simulink model "DvrSimKeybdCircuit_cs"  (R2016a)
settings: Solver=ode5  SolverMode=SingleTasking  StartTime=0.0  StopTime=inf  FixedStep=1/1000  RelTol=1e-3
PreLoadFcn:
  | mbxruntime.callbacks.PreLoadFcn(bdroot);
PostLoadFcn:
  | mbxruntime.callbacks.PostLoadFcn(bdroot);
InitFcn:
  | mbxruntime.callbacks.InitFcn(bdroot);
StartFcn:
  | mbxruntime.callbacks.StartFcn(bdroot);
StopFcn:
  | mbxruntime.callbacks.StopFcn(bdroot);
model workspace (MAT data in the model file):
  mbox_table : struct (value not decoded)
  model_closed = 0
  sim_status = 0
undefined symbols (not defined in the file or in its folder): BMotor1, BMotor2, BrkDelayTime, DControlB, Delay1, Delay2, DiscIntNeverNeededParam, IControlB, JMotor1, JMotor2, PControlB, PreScanCarSimLoadFcn, ratioGearF, ratioGearR, TorqDelayTime, Tstep
undefined symbols (not defined in the file): SteeringColumn, SteeringWheel, WheelL0, WheelL1, WheelR0, WheelR1
libraries: simulink x12, simulink_extras x5, MyLib x3, PreScanSimulinkLibrary x3, Solver_SF x2, pil_lib x1, PreScanUsefulBlocks x1
(part 3 of 9)

== system DvrSimKeybdCircuit_cs/Roewe_550_S_Sedan_1/Subsystem1 ==
  CarSimOut : Inport
  Bus Selector : BusSelector  OutputSignals=SprungMass_Pos_Global_x[m] (signal 1),SprungMass_Pos_Global_y[m] (signal 2),SprungMass_Pos_Global_z[m] (signal 3),VehicleCoG_Vx[km/h] (signal 4),VehicleCoG_Vy[km/h] (signal 5),VehicleCoG_Vz[km/h] (signal 6),SprungMass_Angle_Global_Roll[deg] (signal 7),SprungMass_Angle_Global_Pitch[deg] (signal 8),SprungMass_Angle_Global_Yaw[deg] (signal 9),CarSim_Pos_Wheel_FL_x[m] (signal 10),CarSim_Pos_Wheel_FL_y[m] (signal 11),CarSim_Pos_Wheel_FL_z[m] (signal 12),CarSim_Pos_Wheel_FR_x[m] (signal 13),CarSim_Pos_Wheel_FR_y[m] (signal 14),CarSim_Pos_Wheel_FR_z[m] (signal 15),CarSim_Pos_Wheel_RL_x[m] (signal 16),CarSim_Pos_Wheel_RL_y[m] (signal 17),CarSim_Pos_Wheel_RL_Z[m] (signal 18),CarSim_Pos_Wheel_RR_x[m] (signal 19),CarSim_Pos_Wheel_RR_y[m] (signal 20),CarSim_Pos_Wheel_RR_z[m] (signal 21),CarSim_Angle_Wheel_FL_Roll[deg] (signal 22),CarSim_Angle_Wheel_FL_Rot[rev] (signal 23),CarSim_Angle_Wheel_FL_Steer[deg] (signal 24),CarSim_Angle_Wheel_FR_Roll[deg] (signal 25),CarSim_Angle_Wheel_FR_Rot[rev] (signal 26),CarSim_Angle_Wheel_FR_Steer[deg] (signal 27),CarSim_Angle_Wheel_RL_Roll[deg] (signal 28),CarSim_Angle_Wheel_RL_Rot[rev] (signal 29),CarSim_Angle_Wheel_RL_Steer[deg] (signal 30),CarSim_Angle_Wheel_RR_Roll[deg] (signal 31),CarSim_Angle_Wheel_RR_Rot[rev] (signal 32),CarSim_Angle_Wheel_RR_Steer[deg] (signal 33),SteeringWheelAngle[deg] (signal 34),Axle1ReducedSW (signal 35)
  CarSim2PreScanSTATE : Subsystem  Tag=CarSim2PreScanSTATE  mask(CarSim2PreScan:){z0=0.53}
      mask prompts: z0 "PreScan Actor initial COG z-position wrt GLOBAL axis system [m]"
      mask help: This block converts the outputs coming from the CarSim block into consistent PreScan signals.
  CarSim2PreScan_BUS : Subsystem  Tag=CarSim2PreScan_BUS  mask(PreScan block: CarSim to PreScan BUS){TyreRadius=0.44999998807907104, cogZOffset=0}
      mask prompts: TyreRadius "Tyre Radius [m]"; cogZOffset "cog Z offset [m]"
      mask help: CarSim to PreScan BUS selector
      mask Help: eval('openHelp()')
      mask Display: disp('PreScan BUS\nVehicleDynamics')
  CarSim2PreScan_ContactAdapter : Subsystem  Tag=CarSim2PreScan_ContactAdapter  mask{wheelRadius=0.44999998807907104}
      mask prompts: wheelRadius "Wheel radius:"
  Demux : Demux  Outputs=[18 -1]
  Mux : Mux  Inputs=35
  MuxState1 : Subsystem  Tag=mux/State  mask(Empty Dynamics State Block){positioningmode=on, TimeStep=1/1000}
      mask prompts: positioningmode "Positioning Mode"; TimeStep "Auto Assigned: Time Step [s]"
      mask help:
      | Build the state of an actor based on user input.
      | The user can either use positioning mode or dynamics mode.
      | - When using positioning mode the position and orientation of the actor are set directly based on the input. Expected input is relative to the initial position and orientation of the actor. It's also possible to specify the velocity of the actor, though this input isn't used, only passed on.
      | - When using dynamics mode the position input is ignored. Expected input is velocity and orientation. The velocity is relative the current orientation of the actor, while orientation is relative to its initial orientation. The position of the actor is calculated based on the velocity and orientation given.
      settings: DeleteFcn=PreScanBlockDeleteFcn;
  Scope : Scope
  Terminator_1 : Terminator
  State : Outport
  State_BUS : Outport  Port=2
  ContactParams : Outport  Port=3
  wires:
  CarSimOut/1 -> Bus Selector/1
  Bus Selector/4 -> Mux/4  "<VehicleCoG_Vx[km/h] (signal 4)>"
  Bus Selector/1 -> Mux/1  "<SprungMass_Pos_Global_x[m] (signal 1)>"
  Bus Selector/2 -> Mux/2  "<SprungMass_Pos_Global_y[m] (signal 2)>"
  Bus Selector/3 -> Mux/3  "<SprungMass_Pos_Global_z[m] (signal 3)>"
  Bus Selector/24 -> Mux/24  "<CarSim_Angle_Wheel_FL_Steer[deg] (signal 24)>"
  Bus Selector/28 -> Mux/28  "<CarSim_Angle_Wheel_RL_Roll[deg] (signal 28)>"
  Bus Selector/11 -> Mux/11  "<CarSim_Pos_Wheel_FL_y[m] (signal 11)>"
  Bus Selector/10 -> Mux/10  "<CarSim_Pos_Wheel_FL_x[m] (signal 10)>"
  Bus Selector/7 -> Mux/7  "<SprungMass_Angle_Global_Roll[deg] (signal 7)>"
  Bus Selector/26 -> Mux/26  "<CarSim_Angle_Wheel_FR_Rot[rev] (signal 26)>"
  Bus Selector/30 -> Mux/30  "<CarSim_Angle_Wheel_RL_Steer[deg] (signal 30)>"
  Bus Selector/31 -> Mux/31  "<CarSim_Angle_Wheel_RR_Roll[deg] (signal 31)>"
  Bus Selector/16 -> Mux/16  "<CarSim_Pos_Wheel_RL_x[m] (signal 16)>"
  Bus Selector/6 -> Mux/6  "<VehicleCoG_Vz[km/h] (signal 6)>"
  Bus Selector/12 -> Mux/12  "<CarSim_Pos_Wheel_FL_z[m] (signal 12)>"
  Bus Selector/21 -> Mux/21  "<CarSim_Pos_Wheel_RR_z[m] (signal 21)>"
  Bus Selector/27 -> Mux/27  "<CarSim_Angle_Wheel_FR_Steer[deg] (signal 27)>"
  Bus Selector/5 -> Mux/5  "<VehicleCoG_Vy[km/h] (signal 5)>"
  Bus Selector/19 -> Mux/19  "<CarSim_Pos_Wheel_RR_x[m] (signal 19)>"
  Bus Selector/23 -> Mux/23  "<CarSim_Angle_Wheel_FL_Rot[rev] (signal 23)>"
  Bus Selector/32 -> Mux/32  "<CarSim_Angle_Wheel_RR_Rot[rev] (signal 32)>"
  Bus Selector/29 -> Mux/29  "<CarSim_Angle_Wheel_RL_Rot[rev] (signal 29)>"
  Bus Selector/35 -> Mux/35  "<Axle1ReducedSW (signal 35)>"
  Bus Selector/13 -> Mux/13  "<CarSim_Pos_Wheel_FR_x[m] (signal 13)>"
  Bus Selector/34 -> Mux/34  "<SteeringWheelAngle[deg] (signal 34)>"
  Bus Selector/9 -> Mux/9  "<SprungMass_Angle_Global_Yaw[deg] (signal 9)>"
  Bus Selector/20 -> Mux/20  "<CarSim_Pos_Wheel_RR_y[m] (signal 20)>"
  Bus Selector/25 -> Mux/25  "<CarSim_Angle_Wheel_FR_Roll[deg] (signal 25)>"
  Bus Selector/8 -> Mux/8  "<SprungMass_Angle_Global_Pitch[deg] (signal 8)>"
  Bus Selector/15 -> Mux/15  "<CarSim_Pos_Wheel_FR_z[m] (signal 15)>"
  Bus Selector/17 -> Mux/17  "<CarSim_Pos_Wheel_RL_y[m] (signal 17)>"
  Bus Selector/18 -> Mux/18  "<CarSim_Pos_Wheel_RL_Z[m] (signal 18)>"
  Bus Selector/14 -> Mux/14  "<CarSim_Pos_Wheel_FR_y[m] (signal 14)>"
  Bus Selector/22 -> Mux/22  "<CarSim_Angle_Wheel_FL_Roll[deg] (signal 22)>"
  Bus Selector/33 -> Mux/33  "<CarSim_Angle_Wheel_RR_Steer[deg] (signal 33)>"
  Mux/1 -> CarSim2PreScan_BUS/1(CarSim_In), Demux/1
  MuxState1/1(state) -> CarSim2PreScan_ContactAdapter/1(State), State/1
  CarSim2PreScanSTATE/1(x [m]) -> MuxState1/1(x [m])
  CarSim2PreScanSTATE/2(y [m]) -> MuxState1/2(y [m])
  CarSim2PreScanSTATE/3(z [m]) -> Scope/1, MuxState1/3(z [m])
  CarSim2PreScanSTATE/4(dx [m/s]) -> MuxState1/4(dx [m/s])
  CarSim2PreScanSTATE/5(dy [m/s]) -> MuxState1/5(dy [m/s])
  CarSim2PreScanSTATE/6(dz [m/s]) -> MuxState1/6(dz [m/s])
  CarSim2PreScanSTATE/7(R [rad]) -> MuxState1/7(R [rad])
  CarSim2PreScanSTATE/8(P [rad]) -> MuxState1/8(P [rad])
  CarSim2PreScanSTATE/9(Y [rad]) -> MuxState1/9(Y [rad])
  CarSim2PreScan_BUS/1(PreScanBUS_VehicleDynamics) -> CarSim2PreScan_ContactAdapter/2(State_Bus), State_BUS/1
  CarSim2PreScan_ContactAdapter/1(ContactParams) -> ContactParams/1
  Demux/1 -> CarSim2PreScanSTATE/1(CarSim_In)
  Demux/2 -> Terminator_1/1

== system DvrSimKeybdCircuit_cs/Roewe_550_S_Sedan_1/TIS_1_StandardCoh_Demux ==
  TIS : Inport
  Bus Creator : BusCreator  Inputs=16
  Bus Selector : BusSelector  OutputSignals=ActiveBeamID[-],Range[m],DopplerVelocity[ms-1],DopplerVelocityX[ms-1],DopplerVelocityY[ms-1],DopplerVelocityZ[ms-1],Theta[deg],Phi[deg],TargetID[-],TargetTypeID[-],DopplerVelocityTranslationX[ms-1],DopplerVelocityTranslationY[ms-1],DopplerVelocityTranslationZ[ms-1],DopplerVelocityRotationX[ms-1],DopplerVelocityRotationY[ms-1],DopplerVelocityRotationZ[ms-1]
  ScannerSensorLegacyBusConversion : PreScanUsefulBlocks/ScannerSensorLegacyBusConversion  MAXMESSAGES=MAXMESSAGES
  Out1 : Outport
  Out2 : Outport  Port=2
  Out3 : Outport  Port=3
  Out4 : Outport  Port=4
  Out5 : Outport  Port=5
  Out7 : Outport  Port=6
  Out6 : Outport  Port=7
  wires:
  Bus Selector/16 -> Bus Creator/16  "<DopplerVelocityRotationZ[ms-1]>"
  Bus Selector/15 -> Bus Creator/15  "<DopplerVelocityRotationY[ms-1]>"
  Bus Selector/14 -> Bus Creator/14  "<DopplerVelocityRotationX[ms-1]>"
  Bus Selector/13 -> Bus Creator/13  "<DopplerVelocityTranslationZ[ms-1]>"
  Bus Selector/12 -> Bus Creator/12  "<DopplerVelocityTranslationY[ms-1]>"
  Bus Selector/11 -> Bus Creator/11  "<DopplerVelocityTranslationX[ms-1]>"
  ScannerSensorLegacyBusConversion/1 -> Bus Selector/1
  TIS/1 -> ScannerSensorLegacyBusConversion/1
  Bus Creator/1 -> Out6/1
  Bus Selector/10 -> Bus Creator/10  "<TargetTypeID[-]>"
  Bus Selector/9 -> Out7/1, Bus Creator/9  "<TargetID[-]>"
  Bus Selector/1 -> Out1/1, Bus Creator/1  "<ActiveBeamID[-]>"
  Bus Selector/2 -> Out2/1, Bus Creator/2  "<Range[m]>"
  Bus Selector/7 -> Out4/1, Bus Creator/7  "<Theta[deg]>"
  Bus Selector/8 -> Bus Creator/8, Out5/1  "<Phi[deg]>"
  Bus Selector/3 -> Bus Creator/3, Out3/1  "<DopplerVelocity[ms-1]>"
  Bus Selector/4 -> Bus Creator/4  "<DopplerVelocityX[ms-1]>"
  Bus Selector/5 -> Bus Creator/5  "<DopplerVelocityY[ms-1]>"
  Bus Selector/6 -> Bus Creator/6  "<DopplerVelocityZ[ms-1]>"

== system DvrSimKeybdCircuit_cs/Roewe_550_S_Sedan_1/WheelDisplacement_Mux ==
  Steering Angle Front [rad] : Inport  Tag=inport/JointGroup  SampleTime=50/1000  BusOutputAsStruct=on
  Steering Angle Rear [rad] : Inport  Tag=inport/JointGroup  Port=2  SampleTime=50/1000  BusOutputAsStruct=on
  Rotation [rad] : Inport  Tag=inport/JointGroup  Port=3  SampleTime=50/1000  BusOutputAsStruct=on
  zDisp FL [m] : Inport  Tag=inport/JointGroup  Port=4  SampleTime=50/1000  BusOutputAsStruct=on
  zDisp FR [m] : Inport  Tag=inport/JointGroup  Port=5  SampleTime=50/1000  BusOutputAsStruct=on
  zDisp RL [m] : Inport  Tag=inport/JointGroup  Port=6  SampleTime=50/1000  BusOutputAsStruct=on
  zDisp RR [m] : Inport  Tag=inport/JointGroup  Port=7  SampleTime=50/1000  BusOutputAsStruct=on
  Ground_{1..12} (12 alike) : Ground
  WheelL0_Mux : Subsystem  Tag=mux/Joint  mask(PreScan Mux Block){DisplayName=WheelL0}
      mask prompts: DisplayName "Display Name"
      mask help:
      | This block simulates a generic joint used for generic models. This joint can be enabled/disabled from the GUI.
      |
      | For more information, please click Help.
      settings: DeleteFcn=PreScanBlockDeleteFcn;
      mask Help: eval('openHelp(254)')
  WheelL1_Mux : Subsystem  Tag=mux/Joint  mask(PreScan Mux Block){DisplayName=WheelL1}
      mask prompts: DisplayName "Display Name"
      mask help:
      | This block simulates a generic joint used for generic models. This joint can be enabled/disabled from the GUI.
      |
      | For more information, please click Help.
      settings: DeleteFcn=PreScanBlockDeleteFcn;
      mask Help: eval('openHelp(254)')
  WheelR0_Mux : Subsystem  Tag=mux/Joint  mask(PreScan Mux Block){DisplayName=WheelR0}
      mask prompts: DisplayName "Display Name"
      mask help:
      | This block simulates a generic joint used for generic models. This joint can be enabled/disabled from the GUI.
      |
      | For more information, please click Help.
      settings: DeleteFcn=PreScanBlockDeleteFcn;
      mask Help: eval('openHelp(254)')
  WheelR1_Mux : Subsystem  Tag=mux/Joint  mask(PreScan Mux Block){DisplayName=WheelR1}
      mask prompts: DisplayName "Display Name"
      mask help:
      | This block simulates a generic joint used for generic models. This joint can be enabled/disabled from the GUI.
      |
      | For more information, please click Help.
      settings: DeleteFcn=PreScanBlockDeleteFcn;
      mask Help: eval('openHelp(254)')
  WheelL0_Roewe_550_S_Sedan_1 : Outport  Tag=outport/JointActuator  OutDataTypeStr=Bus: PRESCAN_POSE_DATA  SampleTime=50/1000
  WheelL1_Roewe_550_S_Sedan_1 : Outport  Tag=outport/JointActuator  Port=2  OutDataTypeStr=Bus: PRESCAN_POSE_DATA  SampleTime=50/1000
  WheelR0_Roewe_550_S_Sedan_1 : Outport  Tag=outport/JointActuator  Port=3  OutDataTypeStr=Bus: PRESCAN_POSE_DATA  SampleTime=50/1000
  WheelR1_Roewe_550_S_Sedan_1 : Outport  Tag=outport/JointActuator  Port=4  OutDataTypeStr=Bus: PRESCAN_POSE_DATA  SampleTime=50/1000
  wires:
  WheelL0_Mux/1(Joint) -> WheelL0_Roewe_550_S_Sedan_1/1
  WheelL1_Mux/1(Joint) -> WheelL1_Roewe_550_S_Sedan_1/1
  WheelR0_Mux/1(Joint) -> WheelR0_Roewe_550_S_Sedan_1/1
  WheelR1_Mux/1(Joint) -> WheelR1_Roewe_550_S_Sedan_1/1
  Steering Angle Front [rad]/1 -> WheelR0_Mux/6(Yaw [rad]), WheelL0_Mux/6(Yaw [rad])
  Steering Angle Rear [rad]/1 -> WheelR1_Mux/6(Yaw [rad]), WheelL1_Mux/6(Yaw [rad])
  Rotation [rad]/1 -> WheelR0_Mux/5(Pitch [rad]), WheelL0_Mux/5(Pitch [rad]), WheelR1_Mux/5(Pitch [rad]), WheelL1_Mux/5(Pitch [rad])
  zDisp FL [m]/1 -> WheelL0_Mux/3(Z [m])
  zDisp FR [m]/1 -> WheelR0_Mux/3(Z [m])
  zDisp RL [m]/1 -> WheelL1_Mux/3(Z [m])
  zDisp RR [m]/1 -> WheelR1_Mux/3(Z [m])
  Ground_1/1 -> WheelL0_Mux/1(X [m])
  Ground_2/1 -> WheelL0_Mux/2(Y [m])
  Ground_3/1 -> WheelL0_Mux/4(Roll [rad])
  Ground_4/1 -> WheelL1_Mux/1(X [m])
  Ground_5/1 -> WheelL1_Mux/2(Y [m])
  Ground_6/1 -> WheelL1_Mux/4(Roll [rad])
  Ground_7/1 -> WheelR0_Mux/1(X [m])
  Ground_8/1 -> WheelR0_Mux/2(Y [m])
  Ground_9/1 -> WheelR0_Mux/4(Roll [rad])
  Ground_10/1 -> WheelR1_Mux/1(X [m])
  Ground_11/1 -> WheelR1_Mux/2(Y [m])
  Ground_12/1 -> WheelR1_Mux/4(Roll [rad])

== system DvrSimKeybdCircuit_cs/Roewe_550_S_Sedan_1/d2r SteeringColumn_pivot_Mux ==
  Degrees in : Inport
  Gain1 : Gain  Gain=pi/180  SaturateOnIntegerOverflow=on  OutDataTypeStr=Inherit: Same as input  ParamDataTypeStr=Inherit: Same as input
  Radians out : Outport  InitialOutput=0
  wires:
  Gain1/1 -> Radians out/1
  Degrees in/1 -> Gain1/1

== system DvrSimKeybdCircuit_cs/Roewe_550_S_Sedan_1/d2r SteeringWheel_pivot_Mux ==
  Degrees in : Inport
  Gain1 : Gain  Gain=pi/180  SaturateOnIntegerOverflow=on  OutDataTypeStr=Inherit: Same as input  ParamDataTypeStr=Inherit: Same as input
  Radians out : Outport  InitialOutput=0
  wires:
  Gain1/1 -> Radians out/1
  Degrees in/1 -> Gain1/1

== system DvrSimKeybdCircuit_cs/SteeringColumn_pivot_Roewe_550_S_Sedan_1/Actuator ==
  Joint : Inport
  Bus Selector : BusSelector  OutputSignals=POSITION,ORIENTATION
  visu_Rotate : Subsystem  mask(RPYActuator){UniqueID=UniqueID, Object3DID=Rotate_ObjectID3D, TimeStep=TimeStep}
      mask prompts: UniqueID "Auto-Assigned: Unique ID"; Object3DID "Auto-Assigned: Child 3D Object ID"; TimeStep "Auto-Assigned: Upload Period [s]"
      mask help: Applies angles update to selected child object
      mask Help:
      | Applies position update to selected child object
      | 
      | - UniqueID (double)   : Unique ID of the parent actor
      | - Object3DID (string) : Name of the child 3D object
      mask Display: port_label('input', 1, ['visu_Rotate_' Object3DID])
  visu_Translate : Subsystem  mask(PositionActuator){UniqueID=UniqueID, Object3DID=Translate_ObjectID3D, TimeStep=TimeStep}
      mask prompts: UniqueID "Auto-Assigned: Unique ID"; Object3DID "Auto-Assigned: Child 3D Object ID"; TimeStep "Auto-Assigned: Upload Period [s]"
      mask help: Applies position update to selected child object
      mask Help:
      | Applies position update to selected child object
      | 
      | - UniqueID (double)   : Unique ID of the parent actor
      | - Object3DID (string) : Name of the child 3D object
      mask Display: port_label('input', 1, ['visu_Translate_' Object3DID])
  wires:
  Bus Selector/2 -> visu_Rotate/1(In1)  "<ORIENTATION>"
  Bus Selector/1 -> visu_Translate/1(In1)  "<POSITION>"
  Joint/1 -> Bus Selector/1

== system DvrSimKeybdCircuit_cs/SteeringWheel_pivot_Roewe_550_S_Sedan_1/Actuator ==
  Joint : Inport
  Bus Selector : BusSelector  OutputSignals=POSITION,ORIENTATION
  visu_Rotate : Subsystem  mask(RPYActuator){UniqueID=UniqueID, Object3DID=Rotate_ObjectID3D, TimeStep=TimeStep}
      mask prompts: UniqueID "Auto-Assigned: Unique ID"; Object3DID "Auto-Assigned: Child 3D Object ID"; TimeStep "Auto-Assigned: Upload Period [s]"
      mask help: Applies angles update to selected child object
      mask Help:
      | Applies position update to selected child object
      | 
      | - UniqueID (double)   : Unique ID of the parent actor
      | - Object3DID (string) : Name of the child 3D object
      mask Display: port_label('input', 1, ['visu_Rotate_' Object3DID])
  visu_Translate : Subsystem  mask(PositionActuator){UniqueID=UniqueID, Object3DID=Translate_ObjectID3D, TimeStep=TimeStep}
      mask prompts: UniqueID "Auto-Assigned: Unique ID"; Object3DID "Auto-Assigned: Child 3D Object ID"; TimeStep "Auto-Assigned: Upload Period [s]"
      mask help: Applies position update to selected child object
      mask Help:
      | Applies position update to selected child object
      | 
      | - UniqueID (double)   : Unique ID of the parent actor
      | - Object3DID (string) : Name of the child 3D object
      mask Display: port_label('input', 1, ['visu_Translate_' Object3DID])
  wires:
  Bus Selector/2 -> visu_Rotate/1(In1)  "<ORIENTATION>"
  Bus Selector/1 -> visu_Translate/1(In1)  "<POSITION>"
  Joint/1 -> Bus Selector/1

== system DvrSimKeybdCircuit_cs/WheelL0_Roewe_550_S_Sedan_1/Actuator ==
  Joint : Inport
  Bus Selector : BusSelector  OutputSignals=POSITION,ORIENTATION
  visu_Rotate : Subsystem  mask(RPYActuator){UniqueID=UniqueID, Object3DID=Rotate_ObjectID3D, TimeStep=TimeStep}
      mask prompts: UniqueID "Auto-Assigned: Unique ID"; Object3DID "Auto-Assigned: Child 3D Object ID"; TimeStep "Auto-Assigned: Upload Period [s]"
      mask help: Applies angles update to selected child object
      mask Help:
      | Applies position update to selected child object
      | 
      | - UniqueID (double)   : Unique ID of the parent actor
      | - Object3DID (string) : Name of the child 3D object
      mask Display: port_label('input', 1, ['visu_Rotate_' Object3DID])
  visu_Translate : Subsystem  mask(PositionActuator){UniqueID=UniqueID, Object3DID=Translate_ObjectID3D, TimeStep=TimeStep}
      mask prompts: UniqueID "Auto-Assigned: Unique ID"; Object3DID "Auto-Assigned: Child 3D Object ID"; TimeStep "Auto-Assigned: Upload Period [s]"
      mask help: Applies position update to selected child object
      mask Help:
      | Applies position update to selected child object
      | 
      | - UniqueID (double)   : Unique ID of the parent actor
      | - Object3DID (string) : Name of the child 3D object
      mask Display: port_label('input', 1, ['visu_Translate_' Object3DID])
  wires:
  Bus Selector/2 -> visu_Rotate/1(In1)  "<ORIENTATION>"
  Bus Selector/1 -> visu_Translate/1(In1)  "<POSITION>"
  Joint/1 -> Bus Selector/1

== system DvrSimKeybdCircuit_cs/WheelL1_Roewe_550_S_Sedan_1/Actuator ==
  Joint : Inport
  Bus Selector : BusSelector  OutputSignals=POSITION,ORIENTATION
  visu_Rotate : Subsystem  mask(RPYActuator){UniqueID=UniqueID, Object3DID=Rotate_ObjectID3D, TimeStep=TimeStep}
      mask prompts: UniqueID "Auto-Assigned: Unique ID"; Object3DID "Auto-Assigned: Child 3D Object ID"; TimeStep "Auto-Assigned: Upload Period [s]"
      mask help: Applies angles update to selected child object
      mask Help:
      | Applies position update to selected child object
      | 
      | - UniqueID (double)   : Unique ID of the parent actor
      | - Object3DID (string) : Name of the child 3D object
      mask Display: port_label('input', 1, ['visu_Rotate_' Object3DID])
  visu_Translate : Subsystem  mask(PositionActuator){UniqueID=UniqueID, Object3DID=Translate_ObjectID3D, TimeStep=TimeStep}
      mask prompts: UniqueID "Auto-Assigned: Unique ID"; Object3DID "Auto-Assigned: Child 3D Object ID"; TimeStep "Auto-Assigned: Upload Period [s]"
      mask help: Applies position update to selected child object
      mask Help:
      | Applies position update to selected child object
      | 
      | - UniqueID (double)   : Unique ID of the parent actor
      | - Object3DID (string) : Name of the child 3D object
      mask Display: port_label('input', 1, ['visu_Translate_' Object3DID])
  wires:
  Bus Selector/2 -> visu_Rotate/1(In1)  "<ORIENTATION>"
  Bus Selector/1 -> visu_Translate/1(In1)  "<POSITION>"
  Joint/1 -> Bus Selector/1

== system DvrSimKeybdCircuit_cs/WheelR0_Roewe_550_S_Sedan_1/Actuator ==
  Joint : Inport
  Bus Selector : BusSelector  OutputSignals=POSITION,ORIENTATION
  visu_Rotate : Subsystem  mask(RPYActuator){UniqueID=UniqueID, Object3DID=Rotate_ObjectID3D, TimeStep=TimeStep}
      mask prompts: UniqueID "Auto-Assigned: Unique ID"; Object3DID "Auto-Assigned: Child 3D Object ID"; TimeStep "Auto-Assigned: Upload Period [s]"
      mask help: Applies angles update to selected child object
      mask Help:
      | Applies position update to selected child object
      | 
      | - UniqueID (double)   : Unique ID of the parent actor
      | - Object3DID (string) : Name of the child 3D object
      mask Display: port_label('input', 1, ['visu_Rotate_' Object3DID])
  visu_Translate : Subsystem  mask(PositionActuator){UniqueID=UniqueID, Object3DID=Translate_ObjectID3D, TimeStep=TimeStep}
      mask prompts: UniqueID "Auto-Assigned: Unique ID"; Object3DID "Auto-Assigned: Child 3D Object ID"; TimeStep "Auto-Assigned: Upload Period [s]"
      mask help: Applies position update to selected child object
      mask Help:
      | Applies position update to selected child object
      | 
      | - UniqueID (double)   : Unique ID of the parent actor
      | - Object3DID (string) : Name of the child 3D object
      mask Display: port_label('input', 1, ['visu_Translate_' Object3DID])
  wires:
  Bus Selector/2 -> visu_Rotate/1(In1)  "<ORIENTATION>"
  Bus Selector/1 -> visu_Translate/1(In1)  "<POSITION>"
  Joint/1 -> Bus Selector/1

== system DvrSimKeybdCircuit_cs/WheelR1_Roewe_550_S_Sedan_1/Actuator ==
  Joint : Inport
  Bus Selector : BusSelector  OutputSignals=POSITION,ORIENTATION
  visu_Rotate : Subsystem  mask(RPYActuator){UniqueID=UniqueID, Object3DID=Rotate_ObjectID3D, TimeStep=TimeStep}
      mask prompts: UniqueID "Auto-Assigned: Unique ID"; Object3DID "Auto-Assigned: Child 3D Object ID"; TimeStep "Auto-Assigned: Upload Period [s]"
      mask help: Applies angles update to selected child object
      mask Help:
      | Applies position update to selected child object
      | 
      | - UniqueID (double)   : Unique ID of the parent actor
      | - Object3DID (string) : Name of the child 3D object
      mask Display: port_label('input', 1, ['visu_Rotate_' Object3DID])
  visu_Translate : Subsystem  mask(PositionActuator){UniqueID=UniqueID, Object3DID=Translate_ObjectID3D, TimeStep=TimeStep}
      mask prompts: UniqueID "Auto-Assigned: Unique ID"; Object3DID "Auto-Assigned: Child 3D Object ID"; TimeStep "Auto-Assigned: Upload Period [s]"
      mask help: Applies position update to selected child object
      mask Help:
      | Applies position update to selected child object
      | 
      | - UniqueID (double)   : Unique ID of the parent actor
      | - Object3DID (string) : Name of the child 3D object
      mask Display: port_label('input', 1, ['visu_Translate_' Object3DID])
  wires:
  Bus Selector/2 -> visu_Rotate/1(In1)  "<ORIENTATION>"
  Bus Selector/1 -> visu_Translate/1(In1)  "<POSITION>"
  Joint/1 -> Bus Selector/1

== system DvrSimKeybdCircuit_cs/Roewe_550_S_Sedan_1/AIR_1_Demux/Activate_Switch ==
  BeamID : Inport
  Heading : Inport  Port=2
  Constant : Constant  Value=0
  Product1 : Product  RndMeth=Zero
  Relational Operator : RelationalOperator  Operator=~=  OutDataTypeStr=boolean
  On/Off : Outport
  wires:
  Constant/1 -> Relational Operator/1
  Relational Operator/1 -> Product1/1
  BeamID/1 -> Relational Operator/2
  Product1/1 -> On/Off/1
  Heading/1 -> Product1/2

== system DvrSimKeybdCircuit_cs/Roewe_550_S_Sedan_1/AIR_1_Demux/Signal2ArrayOfSignals1 ==
  note: Set mask parameter VECTORLENGTH
      |  to MAXMESSAGES
  note: Initial state of Previous vector block
      | set to zeros(VECTORLENGTH,1)
  LoopIndex : Inport
  Element : Inport  Port=2
  Assignment : Assignment  IndexOptions=Index vector (port)  Indices=1  OutputSizes=1
  Previous vector : Memory  X0=zeros(VECTORLENGTH,1)  InheritSampleTime=on
  ArrayofElements : Outport
  wires:
  Element/1 -> Assignment/2
  LoopIndex/1 -> Assignment/3
  Previous vector/1 -> Assignment/1
  Assignment/1 -> ArrayofElements/1, Previous vector/1

== system DvrSimKeybdCircuit_cs/Roewe_550_S_Sedan_1/AIR_1_Demux/Signal2ArrayOfSignals2 ==
  note: Set mask parameter VECTORLENGTH
      |  to MAXMESSAGES
  note: Initial state of Previous vector block
      | set to zeros(VECTORLENGTH,1)
  LoopIndex : Inport
  Element : Inport  Port=2
  Assignment : Assignment  IndexOptions=Index vector (port)  Indices=1  OutputSizes=1
  Previous vector : Memory  X0=zeros(VECTORLENGTH,1)  InheritSampleTime=on
  ArrayofElements : Outport
  wires:
  Element/1 -> Assignment/2
  LoopIndex/1 -> Assignment/3
  Previous vector/1 -> Assignment/1
  Assignment/1 -> ArrayofElements/1, Previous vector/1

== system DvrSimKeybdCircuit_cs/Roewe_550_S_Sedan_1/AIR_1_Demux/Signal2ArrayOfSignals3 ==
  note: Set mask parameter VECTORLENGTH
      |  to MAXMESSAGES
  note: Initial state of Previous vector block
      | set to zeros(VECTORLENGTH,1)
  LoopIndex : Inport
  Element : Inport  Port=2
  Assignment : Assignment  IndexOptions=Index vector (port)  Indices=1  OutputSizes=1
  Previous vector : Memory  X0=zeros(VECTORLENGTH,1)  InheritSampleTime=on
  ArrayofElements : Outport
  wires:
  Element/1 -> Assignment/2
  LoopIndex/1 -> Assignment/3
  Previous vector/1 -> Assignment/1
  Assignment/1 -> ArrayofElements/1, Previous vector/1

== system DvrSimKeybdCircuit_cs/Roewe_550_S_Sedan_1/AIR_1_Demux/Signal2ArrayOfSignals4 ==
  note: Set mask parameter VECTORLENGTH
      |  to MAXMESSAGES
  note: Initial state of Previous vector block
      | set to zeros(VECTORLENGTH,1)
  LoopIndex : Inport
  Element : Inport  Port=2
  Assignment : Assignment  IndexOptions=Index vector (port)  Indices=1  OutputSizes=1
  Previous vector : Memory  X0=zeros(VECTORLENGTH,1)  InheritSampleTime=on
  ArrayofElements : Outport
  wires:
  Element/1 -> Assignment/2
  LoopIndex/1 -> Assignment/3
  Previous vector/1 -> Assignment/1
  Assignment/1 -> ArrayofElements/1, Previous vector/1

== system DvrSimKeybdCircuit_cs/Roewe_550_S_Sedan_1/AIR_1_Demux/Signal2ArrayOfSignals5 ==
  note: Set mask parameter VECTORLENGTH
      |  to MAXMESSAGES
  note: Initial state of Previous vector block
      | set to zeros(VECTORLENGTH,1)
  LoopIndex : Inport
  Element : Inport  Port=2
  Assignment : Assignment  IndexOptions=Index vector (port)  Indices=1  OutputSizes=1
  Previous vector : Memory  X0=zeros(VECTORLENGTH,1)  InheritSampleTime=on
  ArrayofElements : Outport
  wires:
  Element/1 -> Assignment/2
  LoopIndex/1 -> Assignment/3
  Previous vector/1 -> Assignment/1
  Assignment/1 -> ArrayofElements/1, Previous vector/1

== system DvrSimKeybdCircuit_cs/Roewe_550_S_Sedan_1/AIR_1_Demux/Signal2ArrayOfSignals6 ==
  note: Set mask parameter VECTORLENGTH
      |  to MAXMESSAGES
  note: Initial state of Previous vector block
      | set to zeros(VECTORLENGTH,1)
  LoopIndex : Inport
  Element : Inport  Port=2
  Assignment : Assignment  IndexOptions=Index vector (port)  Indices=1  OutputSizes=1
  Previous vector : Memory  X0=zeros(VECTORLENGTH,1)  InheritSampleTime=on
  ArrayofElements : Outport
  wires:
  Element/1 -> Assignment/2
  LoopIndex/1 -> Assignment/3
  Previous vector/1 -> Assignment/1
  Assignment/1 -> ArrayofElements/1, Previous vector/1

== system DvrSimKeybdCircuit_cs/Roewe_550_S_Sedan_1/CarSim I//O/ACCAEB ==
  ACCAEBIn : Inport  OutDataTypeStr=Bus: AccAebInputs  BusOutputAsStruct=on
  ACCAEB_sfcn : pil_lib/PIL Block  SimulationMode=SIL  IsTopModelPIL=off  CodeDir=D:\Temp\SimCodeGen\Dest\ACCAEB_ert_rtw  ConfigName=Software-in-the-Loop (SIL)
  __InputSSForSFun__ : Subsystem
  __OutputSSForSFun__ : Subsystem
  ACCAEBOut : Outport
  wires:
  ACCAEBIn/1 -> __InputSSForSFun__/1(ACCAEBIn)
  __InputSSForSFun__/1(__UniqueOutportName__1__) -> ACCAEB_sfcn/1
  ACCAEB_sfcn/1 -> __OutputSSForSFun__/1(__UniqueInportName__1__)
  ACCAEB_sfcn/2 -> __OutputSSForSFun__/2(__UniqueInportName__2__)
  ACCAEB_sfcn/3 -> __OutputSSForSFun__/3(__UniqueInportName__3__)
  ACCAEB_sfcn/4 -> __OutputSSForSFun__/4(__UniqueInportName__4__)
  ACCAEB_sfcn/5 -> __OutputSSForSFun__/5(__UniqueInportName__5__)
  ACCAEB_sfcn/6 -> __OutputSSForSFun__/6(__UniqueInportName__6__)
  ACCAEB_sfcn/7 -> __OutputSSForSFun__/7(__UniqueInportName__7__)
  ACCAEB_sfcn/8 -> __OutputSSForSFun__/8(__UniqueInportName__8__)
  ACCAEB_sfcn/9 -> __OutputSSForSFun__/9(__UniqueInportName__9__)
  ACCAEB_sfcn/10 -> __OutputSSForSFun__/10(__UniqueInportName__10__)
  ACCAEB_sfcn/11 -> __OutputSSForSFun__/11(__UniqueInportName__11__)
  ACCAEB_sfcn/12 -> __OutputSSForSFun__/12(__UniqueInportName__12__)
  ACCAEB_sfcn/13 -> __OutputSSForSFun__/13(__UniqueInportName__13__)
  ACCAEB_sfcn/14 -> __OutputSSForSFun__/14(__UniqueInportName__14__)
  ACCAEB_sfcn/15 -> __OutputSSForSFun__/15(__UniqueInportName__15__)
  ACCAEB_sfcn/16 -> __OutputSSForSFun__/16(__UniqueInportName__16__)
  ACCAEB_sfcn/17 -> __OutputSSForSFun__/17(__UniqueInportName__17__)
  ACCAEB_sfcn/18 -> __OutputSSForSFun__/18(__UniqueInportName__18__)
  ACCAEB_sfcn/19 -> __OutputSSForSFun__/19(__UniqueInportName__19__)
  ACCAEB_sfcn/20 -> __OutputSSForSFun__/20(__UniqueInportName__20__)
  ACCAEB_sfcn/21 -> __OutputSSForSFun__/21(__UniqueInportName__21__)
  ACCAEB_sfcn/22 -> __OutputSSForSFun__/22(__UniqueInportName__22__)
  ACCAEB_sfcn/23 -> __OutputSSForSFun__/23(__UniqueInportName__23__)
  ACCAEB_sfcn/24 -> __OutputSSForSFun__/24(__UniqueInportName__24__)
  ACCAEB_sfcn/25 -> __OutputSSForSFun__/25(__UniqueInportName__25__)
  ACCAEB_sfcn/26 -> __OutputSSForSFun__/26(__UniqueInportName__26__)
  ACCAEB_sfcn/27 -> __OutputSSForSFun__/27(__UniqueInportName__27__)
  ACCAEB_sfcn/28 -> __OutputSSForSFun__/28(__UniqueInportName__28__)
  ACCAEB_sfcn/29 -> __OutputSSForSFun__/29(__UniqueInportName__29__)
  ACCAEB_sfcn/30 -> __OutputSSForSFun__/30(__UniqueInportName__30__)
  ACCAEB_sfcn/31 -> __OutputSSForSFun__/31(__UniqueInportName__31__)
  ACCAEB_sfcn/32 -> __OutputSSForSFun__/32(__UniqueInportName__32__)
  ACCAEB_sfcn/33 -> __OutputSSForSFun__/33(__UniqueInportName__33__)
  ACCAEB_sfcn/34 -> __OutputSSForSFun__/34(__UniqueInportName__34__)
  ACCAEB_sfcn/35 -> __OutputSSForSFun__/35(__UniqueInportName__35__)
  ACCAEB_sfcn/36 -> __OutputSSForSFun__/36(__UniqueInportName__36__)
  ACCAEB_sfcn/37 -> __OutputSSForSFun__/37(__UniqueInportName__37__)
  ACCAEB_sfcn/38 -> __OutputSSForSFun__/38(__UniqueInportName__38__)
  ACCAEB_sfcn/39 -> __OutputSSForSFun__/39(__UniqueInportName__39__)
  ACCAEB_sfcn/40 -> __OutputSSForSFun__/40(__UniqueInportName__40__)
  ACCAEB_sfcn/41 -> __OutputSSForSFun__/41(__UniqueInportName__41__)
  ACCAEB_sfcn/42 -> __OutputSSForSFun__/42(__UniqueInportName__42__)
  ACCAEB_sfcn/43 -> __OutputSSForSFun__/43(__UniqueInportName__43__)
  ACCAEB_sfcn/44 -> __OutputSSForSFun__/44(__UniqueInportName__44__)
  ACCAEB_sfcn/45 -> __OutputSSForSFun__/45(__UniqueInportName__45__)
  ACCAEB_sfcn/46 -> __OutputSSForSFun__/46(__UniqueInportName__46__)
  ACCAEB_sfcn/47 -> __OutputSSForSFun__/47(__UniqueInportName__47__)
  ACCAEB_sfcn/48 -> __OutputSSForSFun__/48(__UniqueInportName__48__)
  ACCAEB_sfcn/49 -> __OutputSSForSFun__/49(__UniqueInportName__49__)
  ACCAEB_sfcn/50 -> __OutputSSForSFun__/50(__UniqueInportName__50__)
  ACCAEB_sfcn/51 -> __OutputSSForSFun__/51(__UniqueInportName__51__)
  ACCAEB_sfcn/52 -> __OutputSSForSFun__/52(__UniqueInportName__52__)
  ACCAEB_sfcn/53 -> __OutputSSForSFun__/53(__UniqueInportName__53__)
  ACCAEB_sfcn/54 -> __OutputSSForSFun__/54(__UniqueInportName__54__)
  ACCAEB_sfcn/55 -> __OutputSSForSFun__/55(__UniqueInportName__55__)
  ACCAEB_sfcn/56 -> __OutputSSForSFun__/56(__UniqueInportName__56__)
  ACCAEB_sfcn/57 -> __OutputSSForSFun__/57(__UniqueInportName__57__)
  ACCAEB_sfcn/58 -> __OutputSSForSFun__/58(__UniqueInportName__58__)
  ACCAEB_sfcn/59 -> __OutputSSForSFun__/59(__UniqueInportName__59__)
  ACCAEB_sfcn/60 -> __OutputSSForSFun__/60(__UniqueInportName__60__)
  ACCAEB_sfcn/61 -> __OutputSSForSFun__/61(__UniqueInportName__61__)
  ACCAEB_sfcn/62 -> __OutputSSForSFun__/62(__UniqueInportName__62__)
  ACCAEB_sfcn/63 -> __OutputSSForSFun__/63(__UniqueInportName__63__)
  ACCAEB_sfcn/64 -> __OutputSSForSFun__/64(__UniqueInportName__64__)
  ACCAEB_sfcn/65 -> __OutputSSForSFun__/65(__UniqueInportName__65__)
  ACCAEB_sfcn/66 -> __OutputSSForSFun__/66(__UniqueInportName__66__)
  ACCAEB_sfcn/67 -> __OutputSSForSFun__/67(__UniqueInportName__67__)
  ACCAEB_sfcn/68 -> __OutputSSForSFun__/68(__UniqueInportName__68__)
  ACCAEB_sfcn/69 -> __OutputSSForSFun__/69(__UniqueInportName__69__)
  ACCAEB_sfcn/70 -> __OutputSSForSFun__/70(__UniqueInportName__70__)
  ACCAEB_sfcn/71 -> __OutputSSForSFun__/71(__UniqueInportName__71__)
  ACCAEB_sfcn/72 -> __OutputSSForSFun__/72(__UniqueInportName__72__)
  ACCAEB_sfcn/73 -> __OutputSSForSFun__/73(__UniqueInportName__73__)
  ACCAEB_sfcn/74 -> __OutputSSForSFun__/74(__UniqueInportName__74__)
  ACCAEB_sfcn/75 -> __OutputSSForSFun__/75(__UniqueInportName__75__)
  ACCAEB_sfcn/76 -> __OutputSSForSFun__/76(__UniqueInportName__76__)
  ACCAEB_sfcn/77 -> __OutputSSForSFun__/77(__UniqueInportName__77__)
  ACCAEB_sfcn/78 -> __OutputSSForSFun__/78(__UniqueInportName__78__)
  ACCAEB_sfcn/79 -> __OutputSSForSFun__/79(__UniqueInportName__79__)
  ACCAEB_sfcn/80 -> __OutputSSForSFun__/80(__UniqueInportName__80__)
  ACCAEB_sfcn/81 -> __OutputSSForSFun__/81(__UniqueInportName__81__)
  ACCAEB_sfcn/82 -> __OutputSSForSFun__/82(__UniqueInportName__82__)
  ACCAEB_sfcn/83 -> __OutputSSForSFun__/83(__UniqueInportName__83__)
  ACCAEB_sfcn/84 -> __OutputSSForSFun__/84(__UniqueInportName__84__)
  ACCAEB_sfcn/85 -> __OutputSSForSFun__/85(__UniqueInportName__85__)
  ACCAEB_sfcn/86 -> __OutputSSForSFun__/86(__UniqueInportName__86__)
  ACCAEB_sfcn/87 -> __OutputSSForSFun__/87(__UniqueInportName__87__)
  ACCAEB_sfcn/88 -> __OutputSSForSFun__/88(__UniqueInportName__88__)
  ACCAEB_sfcn/89 -> __OutputSSForSFun__/89(__UniqueInportName__89__)
  ACCAEB_sfcn/90 -> __OutputSSForSFun__/90(__UniqueInportName__90__)
  ACCAEB_sfcn/91 -> __OutputSSForSFun__/91(__UniqueInportName__91__)
  ACCAEB_sfcn/92 -> __OutputSSForSFun__/92(__UniqueInportName__92__)
  ACCAEB_sfcn/93 -> __OutputSSForSFun__/93(__UniqueInportName__93__)
  ACCAEB_sfcn/94 -> __OutputSSForSFun__/94(__UniqueInportName__94__)
  ACCAEB_sfcn/95 -> __OutputSSForSFun__/95(__UniqueInportName__95__)
  ACCAEB_sfcn/96 -> __OutputSSForSFun__/96(__UniqueInportName__96__)
  ACCAEB_sfcn/97 -> __OutputSSForSFun__/97(__UniqueInportName__97__)
  ACCAEB_sfcn/98 -> __OutputSSForSFun__/98(__UniqueInportName__98__)
  __OutputSSForSFun__/1(ACCAEBOut) -> ACCAEBOut/1
